simulink model "Druga_metoda"  (R2022a)
settings: Solver=VariableStepAuto  StartTime=0.0  StopTime=50  RelTol=1e-3
settings Model: Creator=danie  LastModifiedBy=danie

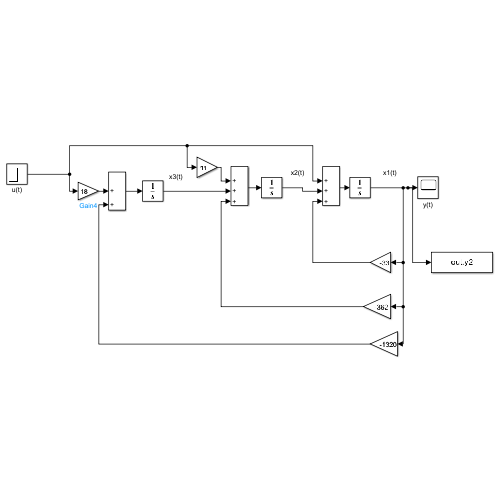
[thumbnail: Simulink's stored preview of the top-level diagram]
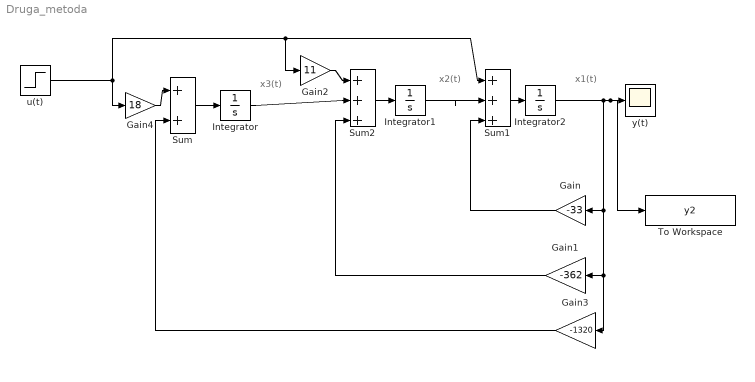
== system Druga_metoda ==
  note: x1(t)
  note: x2(t)
  note: x3(t)
  Gain : Gain  Gain=-33
  Gain1 : Gain  Gain=-362
  Gain2 : Gain  Gain=11
  Gain3 : Gain  Gain=-1320
  Gain4 : Gain  Gain=18
  Integrator : Integrator
  Integrator1 : Integrator
  Integrator2 : Integrator
  Sum : Sum  Inputs=|++
  Sum1 : Sum  Inputs=|+++
  Sum2 : Sum  Inputs=|+++
  To Workspace : ToWorkspace  VariableName=y2  SaveFormat=Structure With Time  SampleTime=-1
  u(t) : Step  SampleTime=0
  y(t) : Scope
  wires:
  Sum/1 -> Integrator/1
  u(t)/1 -> Gain4/1, Sum1/1, Gain2/1
  Integrator2/1 -> Gain3/1, Gain1/1, Gain/1, To Workspace/1, y(t)/1
  Sum1/1 -> Integrator2/1
  Integrator1/1 -> Sum1/2
  Gain/1 -> Sum1/3
  Sum2/1 -> Integrator1/1
  Gain1/1 -> Sum2/3
  Integrator/1 -> Sum2/2
  Gain2/1 -> Sum2/1
  Gain3/1 -> Sum/2
  Gain4/1 -> Sum/1
